simulink model "logger_exec"  (Simulink 3.00)
libraries: execlib x5

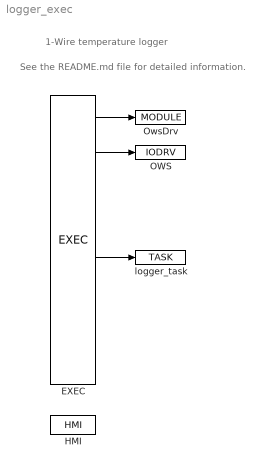
== system logger_exec ==
  note: See the README.md file for detailed information.
  note: 1-Wire temperature logger
  EXEC : execlib/EXEC  target=Generic target device  tick=0.05  ntick0=10  ntick1=50  ntick2=100  ntick3=1200  pri0=5  pri1=9  pri2=13  pri3=18
  HMI : execlib/HMI  IncludeHMI=on  HmiDir=hmi  SourceDir=hmisrc  GenerateWebWatch=on  GenerateRexHMI=on  RedirectToHMI=on  Compression=off
  OWS : execlib/IODRV  module=OwsDrv  classname=OwsDrv  cfgname=ow_cfg.rio  factor=1  stack=10240  pri=3  timer=off
  OwsDrv : execlib/MODULE
  logger_task : execlib/TASK  factor=1  start=0  stop=1  stack=10240  MDLOPEN=on
  wires:
  EXEC/1 -> OwsDrv/1
  EXEC/2 -> OWS/1
  EXEC/5 -> logger_task/1
